simulink model "ssvep_15_electrodes_alone"  (Simulink 6.5)
settings: Solver=FixedStepDiscrete  StartTime=0.0  StopTime=300  FixedStep=1/600  RelTol=1e-3
InitFcn:
  | ssvep_controller_initialization_alone
StopFcn:
  | ssvep_controller_stop_alone
undefined symbols (not defined in the file or in its folder): currentCFG_ssvep_15_electrodes_UA, UA
libraries: Tools x1, dspbuff3 x1, gUSBamplib x1
settings Model: Creator=BMElab  LastModifiedBy=control
settings OptimizationCC: InlineInvariantSignals=on
settings DebuggingCC: MultiTaskDSMMsg=warning  MultiTaskCondExecSysMsg=none  StrictBusMsg=None
settings RTWCC: IncludeERTFirstTime=on

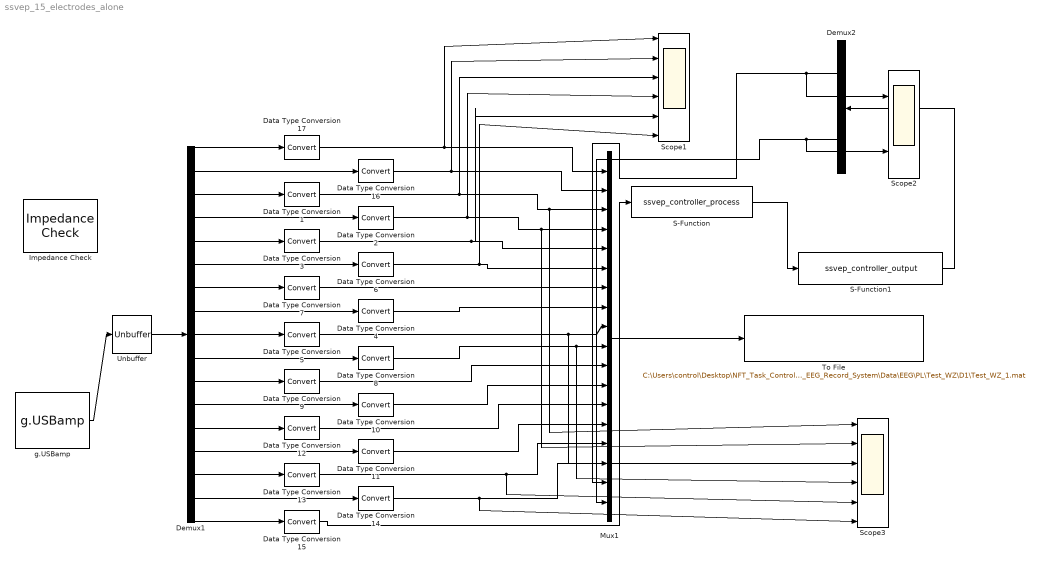
== system ssvep_15_electrodes_alone ==
  Data Type Conversion{1..17} (17 alike) : DataTypeConversion  OutDataTypeMode=double
  Demux1 : Demux  Outputs=17
  Demux2 : Demux  Orientation=left  Outputs=2
  Impedance Check : Tools/Impedance Check  SystemSampleTime=-1
  Mux1 : Mux  Inputs=18
  S-Function : S-Function  FunctionName=ssvep_controller_process
  S-Function1 : S-Function  FunctionName=ssvep_controller_output  Parameters=3,1
  Scope1 : Scope  NumInputPorts=6
      settings: TimeRange=90  YMin=40000~55000~50000~40000~45000~40000  YMax=120000~100000~120000~120000~95000~110000  MaxDataPoints=600000
  Scope2 : Scope  NumInputPorts=2
      settings: TimeRange=60  YMin=-1~0  YMax=1~2  MaxDataPoints=600000
  Scope3 : Scope  NumInputPorts=6
      settings: TimeRange=180  YMin=-1000~-1000~-1000~-1000~-1000~-1000  YMax=1250~1000~1000~1000~1000~1000  SaveName=ScopeData2  MaxDataPoints=3000
  To File : ToFile  Filename=C:\Users\control\Desktop\NFT_Task_Control_and_EEG_Record_System\Data\EEG\PL\Test_WZ\D1\Test_WZ_1.mat  MatrixName=y
  Unbuffer : dspbuff3/Unbuffer  ic=0
  g.USBamp : gUSBamplib/g.USBamp  cfg=currentCFG_ssvep_15_electrodes_UA-2006.09.07.cfg  snr=UA-2006.09.07
  wires:
  g.USBamp/1 -> Unbuffer/1
  Unbuffer/1 -> Demux1/1
  Demux1/9 -> Data Type Conversion5/1
  Demux1/8 -> Data Type Conversion4/1
  Demux1/7 -> Data Type Conversion7/1
  Demux1/6 -> Data Type Conversion6/1
  Demux1/5 -> Data Type Conversion3/1
  Demux1/3 -> Data Type Conversion1/1
  Demux1/4 -> Data Type Conversion2/1
  Demux1/10 -> Data Type Conversion8/1
  Demux1/11 -> Data Type Conversion9/1
  Demux1/12 -> Data Type Conversion10/1
  Demux1/13 -> Data Type Conversion12/1
  Demux1/14 -> Data Type Conversion11/1
  Demux1/15 -> Data Type Conversion13/1
  Demux1/17 -> Data Type Conversion15/1
  Demux1/16 -> Data Type Conversion14/1
  Data Type Conversion2/1 -> Mux1/4, Scope3/2, Scope1/4
  Data Type Conversion1/1 -> Mux1/3, Scope3/1, Scope1/3
  Mux1/1 -> To File/1
  Data Type Conversion3/1 -> Mux1/5, Scope1/5
  Data Type Conversion6/1 -> Mux1/6, Scope1/6
  Data Type Conversion7/1 -> Mux1/7
  Data Type Conversion4/1 -> Mux1/8
  Data Type Conversion5/1 -> Mux1/9, Scope3/3
  Data Type Conversion9/1 -> Mux1/11
  Data Type Conversion10/1 -> Mux1/12
  Data Type Conversion12/1 -> Mux1/13
  Data Type Conversion11/1 -> Mux1/14
  Data Type Conversion13/1 -> Mux1/15, Scope3/5
  Data Type Conversion14/1 -> Mux1/16, Scope3/6
  Demux1/1 -> Data Type Conversion17/1
  Demux1/2 -> Data Type Conversion16/1
  Data Type Conversion16/1 -> Mux1/2, Scope1/2
  Data Type Conversion17/1 -> Mux1/1, Scope1/1
  Data Type Conversion8/1 -> Mux1/10, Scope3/4
  S-Function/1 -> S-Function1/1
  Data Type Conversion15/1 -> S-Function/1
  S-Function1/1 -> Demux2/1
  Demux2/1 -> Mux1/17, Scope2/1
  Demux2/2 -> Mux1/18, Scope2/2
